simulink model "model_sim_CHBjt7"  (R2023b)
settings: Solver=ode3  StartTime=0.0  StopTime=5  FixedStep=01e-6  RelTol=1e-3
InitFcn:
  | sysinit
values from neighbouring files (symbols this model uses):
  C = 0.0234    [sysinit.m]
  f_m = frequency_modulate_start : frequency_modulate_interval : frequency_modulate_end    [simout_chbjt_par.m]    (also in simresjt7.mat = [250 300 350 400 450 500 550 600 650 700 750 800 ... (16 ele)
  L = 0.002    [sysinit.m]
  L_1 = eps    [simout_chb_par.m]    (also in simout_chbjt_par.m; simresjt7.mat = 2.22044604925e-16)
  m = modulate_radio_start : modulate_radio_interval : modulate_radio_end    [simout_chb_par.m]
  R = 1.5    [sysinit.m]
  st = 1e-6    (= 1e-06)    [sysinit.m]
undefined symbols (not defined in the file or in its folder): f, magnitude, Td, Ts2, udc
libraries: spsSeriesRLCBranchLib x120, spsDiodeLib x45, spsIGBTLib x36, spsMeanLib x20, spsCurrentMeasurementLib x16, spsVoltageMeasurementLib x11, spsThreePhaseVIMeasurementLib x10, spsOnDelayLib x9, spsMultiWindingTransformerLib x9, spsUniversalBridgeLib x9, simulink x5, spsRMSLib x2
(part 1 of 3)
settings Model: SimulationMode=accelerator  Creator=Jhchen  LastModifiedBy=ps
settings DataIOCC: ReturnWorkspaceOutputs=off
settings DebuggingCC: RTPrefix=warning

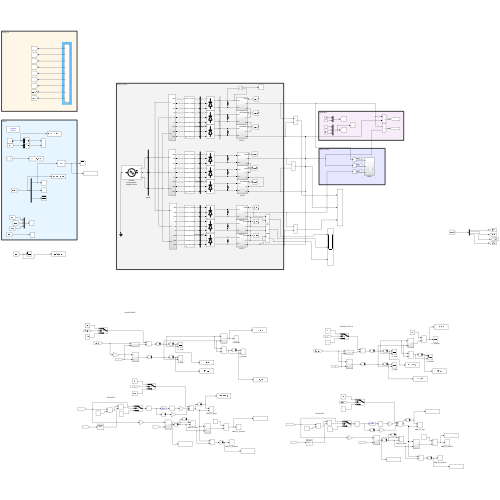
[thumbnail: Simulink's stored preview of the top-level diagram]
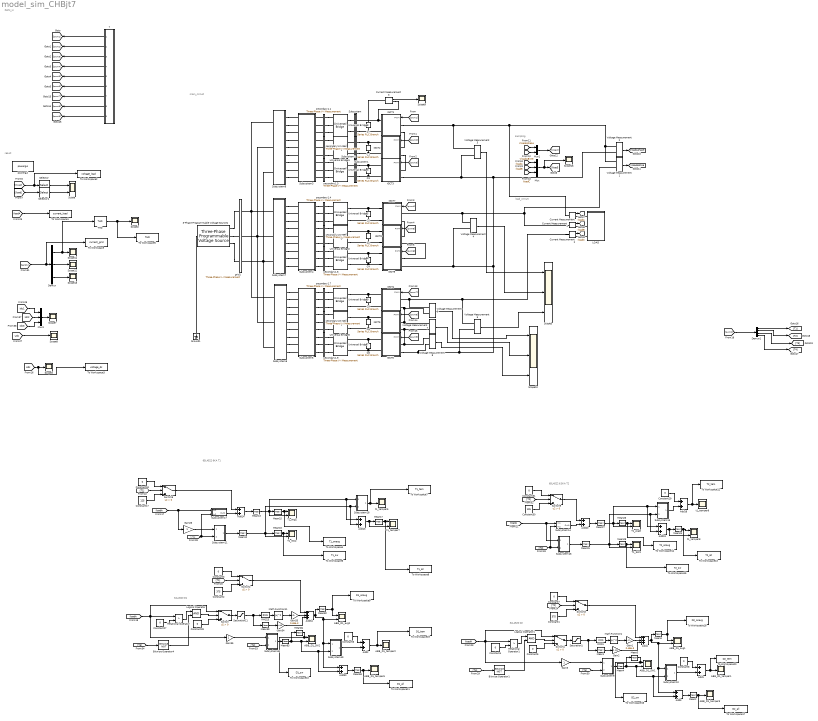
== system model_sim_CHBjt7 ==
  note: load_circuit
  note: main_circuit
  note: PWM_in
  note: result
  note: sampling
  note: 65L4522 6.5KA T2
  note: 34L4520 D1
  note: 34L4520 D2
  note: 65L4522 6KA T1
  3-Phase Programmable Voltage Source1 : spsThreePhaseProgrammableVoltageSourceLib/Three-Phase Programmable Voltage Source  PositiveSequence=[10000 0 50]  VariationEntity=None  VariationType=Step  VariationTypeAlt=Step  VariationStep=0.5  VariationRate=10  VariationMagnitude=0.3  VariationFrequency=2  VariationTiming=[0.05 1]  VariationPhaseA=off  Amplitudes=[1 0.8 1.2 1.0]  TimeValues=[0 0.1 0.15 0.2]  HarmonicGeneration=off  HarmonicA=[5 0.08 -45 2]  HarmonicB=[2 0 0 2]  Timing="[0.1  1]"  BusType=swing  Pref=0  Qref=0  Qmin=-inf  Qmax=inf
  7 : Subsystem  mask{m=m, f=f, f_car=f_m, tt=1/6, ttd=Td}
      mask prompts: m "m_p"; f "f_module"; f_car "f_carrier"; tt "ts"; ttd "td"
      mask DialogControl ParameterGroupVar Prompt: 参数
  ABB_D1_SW1 : Scope  NumInputPorts=2
  ABB_D1_SW2 : Scope  NumInputPorts=2
  ABB_D1_avg1 : Scope  NumInputPorts=2
  ABB_D1_avg2 : Scope  NumInputPorts=2
  ABB_D1_temper{1..3,6} (4 alike) : Scope
  Add{1..3,13..14,18..20,30} (9 alike) : Sum
  Add34 : Sum  Inputs=+++
  Add4 : Sum  Inputs=+++
  Bitwise Operator1 : simulink/Logic and Bit Operations/Bitwise Operator  logicop=NOT  UseBitMask=off  BitMask=bin2dec('11011001')  BitMaskRealWorld=Stored Integer
  Bitwise Operator4 : simulink/Logic and Bit Operations/Bitwise Operator  logicop=NOT  UseBitMask=off  BitMask=bin2dec('11011001')  BitMaskRealWorld=Stored Integer
  C{1..9} (9 alike) : spsSeriesRLCBranchLib/Series RLC Branch  LConnTagsString=__new0  RConnTagsString=__new0  BranchType=C  Resistance=0.0001  Inductance=1.0  SetiL0=off  InitialCurrent=0  Capacitance=C  Setx0=on  InitialVoltage=2500  Measurements=None
  Constant1 : Constant  Value=375
  Constant17 : Constant  Value=125
  Constant{3..8,18,27..29,31} (11 alike) : Constant  Value=0
  Constant2 : Constant  Value=375
  Constant30 : Constant  Value=125
  Current Measurement{,1..3} (4 alike) : spsCurrentMeasurementLib/Current Measurement  PhasorSimulation=off  OutputType=Complex  PSBequivalent=0
  Demux : Demux  Outputs=3
  Demux1 : Demux
  Gain1 : Gain  Gain=0.48e-3
  Gain2 : Gain  Gain=1.46
  Gain26 : Gain
  Gain3 : Gain
  Gain33 : Gain  Gain=0.48e-3
  Gain34 : Gain  Gain=1.46
  Gain35 : Gain
  Ground1 : spsGroundLib/Ground  LConnTagsString=a
  IGCT1 : Subsystem
      settings: PortSchema="{\"entries\":[{\"content\":{\"sides\":[{\"content\":{\"connectorIds\":[\"LConn1\",\"LConn2\"]},\"type\":\"ConnectorPlacement.EquallySpacedRectSide\",\"uuid\":\"ec2238c1-da6e-4f08-8e06-b91b3c8bb0b0\"},{\"content\":{\"connectorIds\":[\"In1\",\"RConn1\",\"RConn2\"],\"side\":\"RIGHT\"},\"type\":\"ConnectorPlacement.EquallySpacedRectSide\",\"uuid\":\"af4a6234-d788-4c0c-860c-0b54063c99a4\"},{\"content\":{\"side\":\"TOP\"},\"type\":\"ConnectorPlacement.EquallySpacedRectSide\",\"uuid\":\"bf1fb326-f044-4e19-8b18-e29d3f1aca1e\"}]},\"type\":\"ConnectorPlacement.EquallySpacedConnector\",\"uuid\":\"a6b09d66-dd31-49c2-be1b-fba678cdcd99\"}],\"packageUris\":[\"http://schema.mathworks.com/mf0/Connector/R2020b\"],\"version\":\"1.0\"}"
  IGCT2 : Subsystem
      settings: PortSchema="{\"entries\":[{\"content\":{\"sides\":[{\"content\":{\"connectorIds\":[\"LConn1\",\"LConn2\"]},\"type\":\"ConnectorPlacement.EquallySpacedRectSide\",\"uuid\":\"3b5227fd-32cc-4097-9a6a-2909540651e9\"},{\"content\":{\"connectorIds\":[\"In1\",\"RConn1\",\"RConn2\"],\"side\":\"RIGHT\"},\"type\":\"ConnectorPlacement.EquallySpacedRectSide\",\"uuid\":\"b0068562-9d9a-456b-acd2-db870c5bcace\"},{\"content\":{\"side\":\"TOP\"},\"type\":\"ConnectorPlacement.EquallySpacedRectSide\",\"uuid\":\"bbecbe08-a8e7-4703-9f6f-443f87d924da\"}]},\"type\":\"ConnectorPlacement.EquallySpacedConnector\",\"uuid\":\"6ec83c7b-e3bb-4502-bc8f-4da9ff103a20\"}],\"packageUris\":[\"http://schema.mathworks.com/mf0/Connector/R2020b\"],\"version\":\"1.0\"}"
  IGCT3 : Subsystem
      settings: PortSchema="{\"entries\":[{\"content\":{\"sides\":[{\"content\":{\"connectorIds\":[\"LConn1\",\"LConn2\"]},\"type\":\"ConnectorPlacement.EquallySpacedRectSide\",\"uuid\":\"3b5227fd-32cc-4097-9a6a-2909540651e9\"},{\"content\":{\"connectorIds\":[\"In1\",\"RConn1\",\"RConn2\"],\"side\":\"RIGHT\"},\"type\":\"ConnectorPlacement.EquallySpacedRectSide\",\"uuid\":\"b0068562-9d9a-456b-acd2-db870c5bcace\"},{\"content\":{\"side\":\"TOP\"},\"type\":\"ConnectorPlacement.EquallySpacedRectSide\",\"uuid\":\"bbecbe08-a8e7-4703-9f6f-443f87d924da\"}]},\"type\":\"ConnectorPlacement.EquallySpacedConnector\",\"uuid\":\"6ec83c7b-e3bb-4502-bc8f-4da9ff103a20\"}],\"packageUris\":[\"http://schema.mathworks.com/mf0/Connector/R2020b\"],\"version\":\"1.0\"}"
  IGCT4 : Subsystem
      settings: PortSchema="{\"entries\":[{\"content\":{\"sides\":[{\"content\":{\"connectorIds\":[\"LConn1\",\"LConn2\"]},\"type\":\"ConnectorPlacement.EquallySpacedRectSide\",\"uuid\":\"ec2238c1-da6e-4f08-8e06-b91b3c8bb0b0\"},{\"content\":{\"connectorIds\":[\"In1\",\"RConn1\",\"RConn2\"],\"side\":\"RIGHT\"},\"type\":\"ConnectorPlacement.EquallySpacedRectSide\",\"uuid\":\"af4a6234-d788-4c0c-860c-0b54063c99a4\"},{\"content\":{\"side\":\"TOP\"},\"type\":\"ConnectorPlacement.EquallySpacedRectSide\",\"uuid\":\"bf1fb326-f044-4e19-8b18-e29d3f1aca1e\"}]},\"type\":\"ConnectorPlacement.EquallySpacedConnector\",\"uuid\":\"a6b09d66-dd31-49c2-be1b-fba678cdcd99\"}],\"packageUris\":[\"http://schema.mathworks.com/mf0/Connector/R2020b\"],\"version\":\"1.0\"}"
  IGCT5 : Subsystem
      settings: PortSchema="{\"entries\":[{\"content\":{\"sides\":[{\"content\":{\"connectorIds\":[\"LConn1\",\"LConn2\"]},\"type\":\"ConnectorPlacement.EquallySpacedRectSide\",\"uuid\":\"3b5227fd-32cc-4097-9a6a-2909540651e9\"},{\"content\":{\"connectorIds\":[\"In1\",\"RConn1\",\"RConn2\"],\"side\":\"RIGHT\"},\"type\":\"ConnectorPlacement.EquallySpacedRectSide\",\"uuid\":\"b0068562-9d9a-456b-acd2-db870c5bcace\"},{\"content\":{\"side\":\"TOP\"},\"type\":\"ConnectorPlacement.EquallySpacedRectSide\",\"uuid\":\"bbecbe08-a8e7-4703-9f6f-443f87d924da\"}]},\"type\":\"ConnectorPlacement.EquallySpacedConnector\",\"uuid\":\"6ec83c7b-e3bb-4502-bc8f-4da9ff103a20\"}],\"packageUris\":[\"http://schema.mathworks.com/mf0/Connector/R2020b\"],\"version\":\"1.0\"}"
  IGCT6 : Subsystem
      settings: PortSchema="{\"entries\":[{\"content\":{\"sides\":[{\"content\":{\"connectorIds\":[\"LConn1\",\"LConn2\"]},\"type\":\"ConnectorPlacement.EquallySpacedRectSide\",\"uuid\":\"3b5227fd-32cc-4097-9a6a-2909540651e9\"},{\"content\":{\"connectorIds\":[\"In1\",\"RConn1\",\"RConn2\"],\"side\":\"RIGHT\"},\"type\":\"ConnectorPlacement.EquallySpacedRectSide\",\"uuid\":\"b0068562-9d9a-456b-acd2-db870c5bcace\"},{\"content\":{\"side\":\"TOP\"},\"type\":\"ConnectorPlacement.EquallySpacedRectSide\",\"uuid\":\"bbecbe08-a8e7-4703-9f6f-443f87d924da\"}]},\"type\":\"ConnectorPlacement.EquallySpacedConnector\",\"uuid\":\"6ec83c7b-e3bb-4502-bc8f-4da9ff103a20\"}],\"packageUris\":[\"http://schema.mathworks.com/mf0/Connector/R2020b\"],\"version\":\"1.0\"}"
  IGCT7 : Subsystem
      settings: PortSchema="{\"entries\":[{\"content\":{\"sides\":[{\"content\":{\"connectorIds\":[\"LConn1\",\"LConn2\"]},\"type\":\"ConnectorPlacement.EquallySpacedRectSide\",\"uuid\":\"ec2238c1-da6e-4f08-8e06-b91b3c8bb0b0\"},{\"content\":{\"connectorIds\":[\"In1\",\"RConn1\",\"RConn2\"],\"side\":\"RIGHT\"},\"type\":\"ConnectorPlacement.EquallySpacedRectSide\",\"uuid\":\"af4a6234-d788-4c0c-860c-0b54063c99a4\"},{\"content\":{\"side\":\"TOP\"},\"type\":\"ConnectorPlacement.EquallySpacedRectSide\",\"uuid\":\"bf1fb326-f044-4e19-8b18-e29d3f1aca1e\"}]},\"type\":\"ConnectorPlacement.EquallySpacedConnector\",\"uuid\":\"a6b09d66-dd31-49c2-be1b-fba678cdcd99\"}],\"packageUris\":[\"http://schema.mathworks.com/mf0/Connector/R2020b\"],\"version\":\"1.0\"}"
  IGCT8 : Subsystem
      settings: PortSchema="{\"entries\":[{\"content\":{\"sides\":[{\"content\":{\"connectorIds\":[\"LConn1\",\"LConn2\"]},\"type\":\"ConnectorPlacement.EquallySpacedRectSide\",\"uuid\":\"3b5227fd-32cc-4097-9a6a-2909540651e9\"},{\"content\":{\"connectorIds\":[\"In1\",\"RConn1\",\"RConn2\"],\"side\":\"RIGHT\"},\"type\":\"ConnectorPlacement.EquallySpacedRectSide\",\"uuid\":\"b0068562-9d9a-456b-acd2-db870c5bcace\"},{\"content\":{\"side\":\"TOP\"},\"type\":\"ConnectorPlacement.EquallySpacedRectSide\",\"uuid\":\"bbecbe08-a8e7-4703-9f6f-443f87d924da\"}]},\"type\":\"ConnectorPlacement.EquallySpacedConnector\",\"uuid\":\"6ec83c7b-e3bb-4502-bc8f-4da9ff103a20\"}],\"packageUris\":[\"http://schema.mathworks.com/mf0/Connector/R2020b\"],\"version\":\"1.0\"}"
  IGCT9 : Subsystem
      settings: PortSchema="{\"entries\":[{\"content\":{\"sides\":[{\"content\":{\"connectorIds\":[\"LConn1\",\"LConn2\"]},\"type\":\"ConnectorPlacement.EquallySpacedRectSide\",\"uuid\":\"3b5227fd-32cc-4097-9a6a-2909540651e9\"},{\"content\":{\"connectorIds\":[\"In1\",\"RConn1\",\"RConn2\"],\"side\":\"RIGHT\"},\"type\":\"ConnectorPlacement.EquallySpacedRectSide\",\"uuid\":\"b0068562-9d9a-456b-acd2-db870c5bcace\"},{\"content\":{\"side\":\"TOP\"},\"type\":\"ConnectorPlacement.EquallySpacedRectSide\",\"uuid\":\"bbecbe08-a8e7-4703-9f6f-443f87d924da\"}]},\"type\":\"ConnectorPlacement.EquallySpacedConnector\",\"uuid\":\"6ec83c7b-e3bb-4502-bc8f-4da9ff103a20\"}],\"packageUris\":[\"http://schema.mathworks.com/mf0/Connector/R2020b\"],\"version\":\"1.0\"}"
  LOAD : Subsystem
  Logical Operator : Logic  AllPortsSameDT=off  OutDataTypeStr=boolean
  Logical Operator1 : Logic  AllPortsSameDT=off  OutDataTypeStr=boolean
  Math Function1 : Math  Operator=magnitude^2  SignedPower=on
  Math Function11 : Math  Operator=magnitude^2  SignedPower=on
  Mean{1,4,12..13,25,27,39,83} (8 alike) : spsMeanLib/Mean  Freq=2000  Vinit=0  Ts=1e-6
  Mean{15..16,26,28} (4 alike) : spsMeanLib/Mean  Freq=f  Vinit=0  Ts=Ts2
  Mean{2..3,5,17,24,58,82,84} (8 alike) : spsMeanLib/Mean  Freq=f  Vinit=0  Ts=1e-6
  Mux : Mux  Inputs=3
  Mux1 : Mux  Inputs=2
  Mux3 : Mux  Inputs=3
  RMS1 : spsRMSLib/RMS  TrueRMS=on  Freq=2000  RMSInit=0  Ts=1e-6
  RMS23 : spsRMSLib/RMS  TrueRMS=on  Freq=2000  RMSInit=0  Ts=1e-6
  Relational Operator : RelationalOperator  Operator=>  OutDataTypeStr=boolean  RndMeth=Simplest  InputSameDT=off
  Relational Operator1 : RelationalOperator  Operator=>  OutDataTypeStr=boolean  RndMeth=Simplest  InputSameDT=off
  Saturation1 : Saturate  UpperLimit=5500  LowerLimit=0
  Saturation11 : Saturate  UpperLimit=5500  LowerLimit=0
  Scope : Scope  NumInputPorts=2
  Scope10 : Scope  NumInputPorts=3
  Scope{2..3,7..9,11..13,16} (9 alike) : Scope
  Scope5 : Scope  NumInputPorts=3
  Selector : Selector  InputPortWidth=2  IndexOptions=Index vector (dialog)  Indices=[1]  OutputSizes=1
  Selector1 : Selector  InputPortWidth=3  IndexOptions=Index vector (dialog)  Indices=[1]  OutputSizes=1
  Subsystem : Subsystem
  Subsystem1 : Subsystem
  Subsystem10 : Subsystem
  Subsystem11 : Subsystem
  Subsystem14 : Subsystem
  Subsystem15 : Subsystem
  Subsystem16 : Subsystem
  Subsystem17 : Subsystem
  Subsystem18 : Subsystem
  Subsystem2 : Subsystem
  Subsystem3 : Subsystem  mask{L_in=L_1}
      mask prompts: L_in "L"
      mask DialogControl ParameterGroupVar Prompt: 参数
  Subsystem4 : Subsystem  mask{L_in=L_1}
      mask prompts: L_in "L"
      mask DialogControl ParameterGroupVar Prompt: 参数
  Subsystem48 : Subsystem
  Subsystem49 : Subsystem
  Subsystem5 : Subsystem  mask{L_in=L_1}
      mask prompts: L_in "L"
      mask DialogControl ParameterGroupVar Prompt: 参数
  Subsystem6 : Subsystem
  Subsystem7 : Subsystem
  Subsystem8 : Subsystem
  Subsystem9 : Subsystem
  Switch{,1..3,6,9} (6 alike) : Switch  Criteria=u2 > Threshold  SaturateOnIntegerOverflow=off  InputSameDT=off
  T1_SW2 : Scope  NumInputPorts=2
  T1_SW3 : Scope  NumInputPorts=2
  T1_avg2 : Scope  NumInputPorts=2
  T1_avg3 : Scope  NumInputPorts=2
  THD : spsTHDLib/THD  Freq=50  Ts=0
  To Workspace : ToWorkspace  VariableName=current_grid  SaveFormat=Structure With Time  SampleTime=-1
  To Workspace1 : ToWorkspace  VariableName=current_load  SaveFormat=Structure With Time  SampleTime=-1
  To Workspace10 : ToWorkspace  VariableName=D1_sw  SaveFormat=Structure With Time  SampleTime=-1
  To Workspace11 : ToWorkspace  VariableName=D1_all  SaveFormat=Structure With Time  SampleTime=-1
  To Workspace12 : ToWorkspace  VariableName=T2_tem  SaveFormat=Structure With Time  SampleTime=-1
  To Workspace13 : ToWorkspace  VariableName=T2_all  SaveFormat=Structure With Time  SampleTime=-1
  To Workspace14 : ToWorkspace  VariableName=T2_onavg  SaveFormat=Structure With Time  SampleTime=-1
  To Workspace15 : ToWorkspace  VariableName=T2_sw  SaveFormat=Structure With Time  SampleTime=-1
  To Workspace16 : ToWorkspace  VariableName=D2_sw  SaveFormat=Structure With Time  SampleTime=-1
  To Workspace17 : ToWorkspace  VariableName=D2_all  SaveFormat=Structure With Time  SampleTime=-1
  To Workspace18 : ToWorkspace  VariableName=D2_onavg  SaveFormat=Structure With Time  SampleTime=-1
  To Workspace19 : ToWorkspace  VariableName=D1_tem  SaveFormat=Structure With Time  SampleTime=-1
  To Workspace2 : ToWorkspace  VariableName=voltage_load  SaveFormat=Structure With Time  SampleTime=-1
  To Workspace20 : ToWorkspace  VariableName=D2_tem  SaveFormat=Structure With Time  SampleTime=-1
  To Workspace3 : ToWorkspace  VariableName=voltage_dc  SaveFormat=Structure With Time  SampleTime=-1
  To Workspace4 : ToWorkspace  VariableName=T1_onavg  SaveFormat=Structure With Time  SampleTime=-1
  To Workspace5 : ToWorkspace  VariableName=THD  SaveFormat=Structure With Time  SampleTime=-1
  To Workspace6 : ToWorkspace  VariableName=T1_sw  SaveFormat=Structure With Time  SampleTime=-1
  To Workspace7 : ToWorkspace  VariableName=T1_tem  SaveFormat=Structure With Time  SampleTime=-1
  To Workspace8 : ToWorkspace  VariableName=T1_all  SaveFormat=Structure With Time  SampleTime=-1
  To Workspace9 : ToWorkspace  VariableName=D1_onavg  SaveFormat=Structure With Time  SampleTime=-1
  Universal Bridge{1..9} (9 alike) : spsUniversalBridgeLib/Universal Bridge  Arms=3  SnubberResistance=1e5  SnubberCapacitance=inf  Device=Diodes  Ron=1e-3  Lon=0  ForwardVoltages="[  0  0  ]"  ForwardVoltage=0  GTOparameters=[ 10e-6 , 20e-6 ]  IGBTparameters=[ 1e-6 , 2e-6 ]  Measurements=None  Measurements_2=None  converterType=Rectifier
  Voltage Measurement{1..8} (8 alike) : spsVoltageMeasurementLib/Voltage Measurement  PhasorSimulation=off  OutputType=Complex  PSBequivalent=0
  grid1 : spsThreePhaseVIMeasurementLib/Three-Phase V-I Measurement  VoltageMeasurement=phase-to-ground  SetLabelV=on  LabelV=Vgrid1  Vpu=off  VpuLL=off  CurrentMeasurement=yes  SetLabelI=on  LabelI=Igrid1  Ipu=off  Pbase=1e3  Vbase=380  OutputType=Magnitude  PhasorSimulation=off  PSBequivalent=0
  powergui : spspowerguiLib/powergui  Priority=1  SimulationMode=Discrete  SampleTime=st  frequency=60  Iterations=50  frequencyindice=50  Pbase=100e6  ErrMax=1e-4  UnitsV=kV  UnitsW=MW  buscounter=0  FunctionMessages=off  echomessages=off  EnableUseOfTLC=off  CurrentSourceSwitches=off  DisableSnubberDevices=off  DisableRonSwitches=off  DisableVfSwitches=off  DisplayEquations=off  AutomaticDiscreteSolvers=off  SolverType=Tustin/Backward Euler (TBE)  Interpol=off  ExternalGateDelay=off  methode=off  Ts=100  x0status=blocks  SPID=on  SwTol=0  HookPort=off  NonlinearTolerance=1e-4  nMaxIteration=100  ContinueOnMaxIteration=off  RestoreLinks=warning  ResistiveCurrentMeasurement=off  Frange=[0:2:500]  Ylog=off  Xlog=on  ShowGrid=off  save=off  variable=ZData  structure=0  ZoomFFT=off  StartTime=0.0  cycles=1  DisplayStyle=1  fundamental=60  FreqAxis=off  MaxFrequency=1000  frequencyindicesteady=1  RmsSteady=1  display=off
  secondary1.1 : spsThreePhaseVIMeasurementLib/Three-Phase V-I Measurement  VoltageMeasurement=phase-to-phase  SetLabelV=on  LabelV=Vsecondary_a1  Vpu=off  VpuLL=off  CurrentMeasurement=yes  SetLabelI=on  LabelI=Isecondary_a1  Ipu=off  Pbase=1e3  Vbase=380  OutputType=Magnitude  PhasorSimulation=off  PSBequivalent=0
  secondary1.2 : spsThreePhaseVIMeasurementLib/Three-Phase V-I Measurement  VoltageMeasurement=phase-to-phase  SetLabelV=on  LabelV=Vsecondary_a2  Vpu=off  VpuLL=off  CurrentMeasurement=yes  SetLabelI=on  LabelI=Isecondary_a2  Ipu=off  Pbase=1e3  Vbase=380  OutputType=Magnitude  PhasorSimulation=off  PSBequivalent=0
  secondary1.3 : spsThreePhaseVIMeasurementLib/Three-Phase V-I Measurement  VoltageMeasurement=phase-to-phase  SetLabelV=on  LabelV=Vsecondary_a3  Vpu=off  VpuLL=off  CurrentMeasurement=yes  SetLabelI=on  LabelI=Isecondary_a3  Ipu=off  Pbase=1e3  Vbase=380  OutputType=Magnitude  PhasorSimulation=off  PSBequivalent=0
  secondary1.4 : spsThreePhaseVIMeasurementLib/Three-Phase V-I Measurement  VoltageMeasurement=phase-to-phase  SetLabelV=on  LabelV=Vsecondary_a4  Vpu=off  VpuLL=off  CurrentMeasurement=yes  SetLabelI=on  LabelI=Isecondary_a4  Ipu=off  Pbase=1e3  Vbase=380  OutputType=Magnitude  PhasorSimulation=off  PSBequivalent=0
  secondary1.5 : spsThreePhaseVIMeasurementLib/Three-Phase V-I Measurement  VoltageMeasurement=phase-to-phase  SetLabelV=on  LabelV=Vsecondary_a5  Vpu=off  VpuLL=off  CurrentMeasurement=yes  SetLabelI=on  LabelI=Isecondary_a5  Ipu=off  Pbase=1e3  Vbase=380  OutputType=Magnitude  PhasorSimulation=off  PSBequivalent=0
  secondary1.6 : spsThreePhaseVIMeasurementLib/Three-Phase V-I Measurement  VoltageMeasurement=phase-to-phase  SetLabelV=on  LabelV=Vsecondary_a6  Vpu=off  VpuLL=off  CurrentMeasurement=yes  SetLabelI=on  LabelI=Isecondary_a6  Ipu=off  Pbase=1e3  Vbase=380  OutputType=Magnitude  PhasorSimulation=off  PSBequivalent=0
  secondary1.7 : spsThreePhaseVIMeasurementLib/Three-Phase V-I Measurement  VoltageMeasurement=phase-to-phase  SetLabelV=on  LabelV=Vsecondary_a7  Vpu=off  VpuLL=off  CurrentMeasurement=yes  SetLabelI=on  LabelI=Isecondary_a7  Ipu=off  Pbase=1e3  Vbase=380  OutputType=Magnitude  PhasorSimulation=off  PSBequivalent=0
  secondary1.8 : spsThreePhaseVIMeasurementLib/Three-Phase V-I Measurement  VoltageMeasurement=phase-to-phase  SetLabelV=on  LabelV=Vsecondary_a8  Vpu=off  VpuLL=off  CurrentMeasurement=yes  SetLabelI=on  LabelI=Isecondary_a8  Ipu=off  Pbase=1e3  Vbase=380  OutputType=Magnitude  PhasorSimulation=off  PSBequivalent=0
  secondary1.9 : spsThreePhaseVIMeasurementLib/Three-Phase V-I Measurement  VoltageMeasurement=phase-to-phase  SetLabelV=on  LabelV=Vsecondary_a9  Vpu=off  VpuLL=off  CurrentMeasurement=yes  SetLabelI=on  LabelI=Isecondary_a9  Ipu=off  Pbase=1e3  Vbase=380  OutputType=Magnitude  PhasorSimulation=off  PSBequivalent=0
  t1_temper5 : Scope
  t1_temper7 : Scope  NumInputPorts=2
  t1_temper8 : Scope  NumInputPorts=2
  t1_temper9 : Scope
  tag scope: IloadA=global, IloadB=global, IloadC=global, VloadABline=global, VloadAphase=global
  wires:
  [pwm1] -> IGCT1/1(PWM)
  [Vload] -> To Workspace2/1, Selector/1
  Selector/1 -> Scope/1
  [Iload] -> Selector1/1
  Selector1/1 -> Scope/2
  Current Measurement/1 -> [IloadA]
  Current Measurement1/1 -> [IloadB]
  Current Measurement2/1 -> [IloadC]
  [IloadC] -> Mux/3
  [IloadB] -> Mux/2
  [IloadA] -> Mux/1
  Mux/1 -> Scope16/1, [Iload]
  Voltage Measurement2/1 -> [VloadAphase]
  Voltage Measurement1/1 -> [VloadABline]
  [VloadAphase] -> Mux1/1
  [VloadABline] -> Mux1/2
  Mux1/1 -> [Vload]
  [Igrid1] -> To Workspace/1, Demux/1
  [IloadA] -> To Workspace1/1
  [pwm4] -> IGCT7/1(PWM)
  [pwm5] -> IGCT8/1(PWM)
  [pwm6] -> IGCT9/1(PWM)
  [pwm7] -> IGCT4/1(PWM)
  [pwm8] -> IGCT5/1(PWM)
  [pwm9] -> IGCT6/1(PWM)
  [pwm2] -> IGCT2/1(PWM)
  [pwm3] -> IGCT3/1(PWM)
  7/1(Out1) -> [pwm1]
  7/2(Out2) -> [pwm2]
  7/3(Out3) -> [pwm3]
  7/9(Out9) -> [pwm9]
  7/8(Out8) -> [pwm8]
  7/7(Out7) -> [pwm7]
  7/6(Out6) -> [pwm6]
  7/5(Out5) -> [pwm5]
  7/4(Out4) -> [pwm4]
  Voltage Measurement5/1 -> Scope5/3
  Voltage Measurement4/1 -> Scope5/2
  Voltage Measurement3/1 -> Scope5/1
  [Udc] -> Scope8/1
  Current Measurement3/1 -> Scope9/1
  Voltage Measurement6/1 -> Scope10/1
  Voltage Measurement7/1 -> Scope10/2
  Voltage Measurement8/1 -> Scope10/3
  Demux/1 -> THD/1, Scope11/1
  Demux/3 -> Scope13/1
  Demux/2 -> Scope12/1
  [Idc1] -> Mux3/1
  [Idc2] -> Mux3/2
  [Idc3] -> Mux3/3
  Mux3/1 -> Scope7/1
  THD/1 -> To Workspace5/1, Scope2/1
  [Udc] -> To Workspace3/1, Scope3/1
  [IloadA] -> Switch/1, Gain35/1, Relational Operator/1
  Mean17/1 -> To Workspace8/1, t1_temper7/1
  Add13/1 -> t1_temper7/2, Mean17/1
  Demux1/1 -> [T1]
  Gain34/1 -> Add34/3
  Constant28/1 -> Switch/3
  Bitwise Operator4/1 -> Logical Operator/2
  Constant17/1 -> Switch6/3
  Constant2/1 -> Switch2/3
  Demux1/2 -> [T2]
  Mean16/1 -> To Workspace6/1, T1_SW2/1
  [T1] -> Switch2/2
  Add34/1 -> Add30/1, Subsystem49/1(In1), ABB_D1_avg2/2, Mean82/1
  Add20/1 -> Mean27/1
  Add19/1 -> t1_temper8/2, Mean24/1
  Gain26/1 -> Subsystem11/1(In1)
  Switch6/1 -> Add14/1
  Mean12/1 -> Subsystem18/2(In2), Add13/2, T1_SW2/2, Mean16/1
  Subsystem17/1(Out1) -> Add14/2
  Add30/1 -> Mean58/1
  Constant6/1 -> Add2/1
  Mean58/1 -> ABB_D1_temper6/1, To Workspace11/1
  Mean28/1 -> To Workspace15/1, T1_SW3/1
  [T1] -> Subsystem11/2(In2), Subsystem17/2(In2)
  [IloadA] -> Gain26/1, Subsystem17/1(In1)
  Add3/1 -> Mean2/1
  [IloadA] -> Subsystem16/1(In1), Subsystem14/1(In1)
  Mean5/1 -> ABB_D1_SW1/1, To Workspace16/1
  RMS1/1 -> Math Function1/1
  Add2/1 -> To Workspace19/1, ABB_D1_temper2/1
  Add4/1 -> Mean3/1, ABB_D1_avg1/2, Subsystem10/1(In1), Add3/1
  Relational Operator1/1 -> Logical Operator1/1
  [T2] -> Switch3/2
  Constant7/1 -> Switch3/1
  Gain1/1 -> Add4/2
  [IloadA] -> Relational Operator1/1, Gain3/1, Switch1/1
  Subsystem11/1(Out1) -> Mean12/1
  Add1/1 -> To Workspace20/1, ABB_D1_temper1/1
  Gain3/1 -> Subsystem9/1(In1)
  Mean3/1 -> To Workspace18/1, ABB_D1_avg1/1
  Demux1/3 -> [T3]
  Logical Operator1/1 -> Switch1/2
  Switch1/1 -> Saturation1/1
  Mean4/1 -> ABB_D1_SW1/2, Subsystem10/2(In2), Add3/2, Mean5/1
  Saturation1/1 -> RMS1/1, Mean1/1
  Add18/1 -> To Workspace12/1, t1_temper9/1
  Constant18/1 -> Switch6/1
  Subsystem16/1(Out1) -> Mean25/1
  Constant29/1 -> Add18/1
  [T2] -> Subsystem14/2(In2), Subsystem16/2(In2)
  Subsystem15/1(Out1) -> Add18/2
  Mean27/1 -> T1_avg3/2, Mean26/1, Subsystem15/1(In1), Add19/1
  Relational Operator/1 -> Logical Operator/1
  Subsystem14/1(Out1) -> Add20/2
  [T1] -> Switch6/2
  Constant31/1 -> Switch9/1
  Constant1/1 -> Switch3/3
  Mean24/1 -> To Workspace13/1, t1_temper8/1
  RMS23/1 -> Math Function11/1
  [T2] -> Switch9/2
  Mean84/1 -> To Workspace10/1, ABB_D1_SW2/1
  Saturation11/1 -> Mean39/1, RMS23/1
  Switch9/1 -> Add20/1
  Constant30/1 -> Switch9/3
  Constant5/1 -> Switch1/3
  Mean25/1 -> Subsystem15/2(In2), Add19/2, T1_SW3/2, Mean28/1
  Mean82/1 -> ABB_D1_avg2/1, To Workspace9/1
  Gain35/1 -> Subsystem48/1(In1)
  Math Function11/1 -> Gain33/1
  Bitwise Operator1/1 -> Logical Operator1/2
  Add14/1 -> Mean13/1
  Mean26/1 -> To Workspace14/1, T1_avg3/1
  Mean39/1 -> Gain34/1
  Switch2/1 -> Add34/1
  Constant27/1 -> Relational Operator/2
  Subsystem48/1(Out1) -> Mean83/1
  Subsystem18/1(Out1) -> To Workspace7/1, t1_temper5/1
  Mean15/1 -> To Workspace4/1, T1_avg2/1
  [T3] -> Subsystem48/2(In2)
  Demux1/4 -> [T4]
  Constant8/1 -> Add1/1
  Gain2/1 -> Add4/3
  Mean13/1 -> T1_avg2/2, Mean15/1, Subsystem18/1(In1), Add13/1
  [T3] -> Bitwise Operator4/1
  [T4] -> Subsystem9/2(In2)
  Subsystem10/1(Out1) -> Add1/2
  Math Function1/1 -> Gain1/1
  Mean2/1 -> To Workspace17/1, ABB_D1_temper3/1
  Subsystem49/1(Out1) -> Add2/2
  [T4] -> Bitwise Operator1/1
  Logical Operator/1 -> Switch/2
  Constant3/1 -> Switch2/1
  Switch/1 -> Saturation11/1
  Constant4/1 -> Relational Operator1/2
  Mean1/1 -> Gain2/1
  [pwm1] -> Demux1/1
  Mean83/1 -> Mean84/1, Add30/2, Subsystem49/2(In2), ABB_D1_SW2/2
  Switch3/1 -> Add4/1
  Subsystem9/1(Out1) -> Mean4/1
  Gain33/1 -> Add34/2
  connections:
  3-Phase Programmable Voltage Source1/RConn3 -- grid1/LConn3
  3-Phase Programmable Voltage Source1/RConn2 -- grid1/LConn2
  secondary1.1/RConn2 -- Universal Bridge8/LConn2
  secondary1.1/RConn3 -- Universal Bridge8/LConn3
  secondary1.2/RConn1 -- Universal Bridge1/LConn1
  secondary1.2/RConn2 -- Universal Bridge1/LConn2
  secondary1.2/RConn3 -- Universal Bridge1/LConn3
  secondary1.1/RConn1 -- Universal Bridge8/LConn1
  IGCT2/LConn2 -- Subsystem1/RConn2 -- C1/RConn1
  IGCT2/LConn1 -- Subsystem1/RConn1 -- C1/LConn1
  Universal Bridge8/RConn1 -- Subsystem/LConn1
  Universal Bridge8/RConn2 -- Subsystem/LConn2
  Subsystem/RConn2 -- IGCT1/LConn2 -- C7/RConn1
  IGCT1/LConn1 -- Current Measurement3/RConn1 -- Subsystem/RConn1
  IGCT1/RConn2 -- IGCT2/RConn1
  IGCT3/LConn2 -- Subsystem2/RConn2 -- C3/RConn1
  secondary1.3/RConn1 -- Universal Bridge3/LConn1
  C3/LConn1 -- Subsystem2/RConn1 -- IGCT3/LConn1
  secondary1.3/RConn3 -- Universal Bridge3/LConn3
  secondary1.3/RConn2 -- Universal Bridge3/LConn2
  3-Phase Programmable Voltage Source1/RConn1 -- grid1/LConn1
  LOAD/LConn2 -- Current Measurement1/RConn1
  Current Measurement/RConn1 -- LOAD/LConn1
  Current Measurement2/RConn1 -- LOAD/LConn3
  Ground1/LConn1 -- 3-Phase Programmable Voltage Source1/LConn1
  IGCT2/RConn2 -- IGCT3/RConn1
  IGCT6/RConn2 -- Voltage Measurement8/LConn2 -- Voltage Measurement5/LConn2 -- Voltage Measurement3/LConn2 -- IGCT3/RConn2 -- Voltage Measurement2/LConn2 -- Voltage Measurement4/LConn2 -- IGCT9/RConn2
  C5/LConn1 -- IGCT7/LConn1 -- Universal Bridge5/RConn1
  C5/RConn1 -- IGCT7/LConn2 -- Universal Bridge5/RConn2
  C4/LConn1 -- IGCT9/LConn1 -- Universal Bridge4/RConn1
  Universal Bridge4/RConn2 -- IGCT9/LConn2 -- C4/RConn1
  Universal Bridge2/RConn2 -- IGCT8/LConn2 -- C2/RConn1
  Universal Bridge2/RConn1 -- IGCT8/LConn1 -- C2/LConn1
  secondary1.6/RConn2 -- Universal Bridge4/LConn2
  secondary1.4/RConn3 -- Universal Bridge5/LConn3
  IGCT9/RConn1 -- IGCT8/RConn2
  secondary1.5/RConn1 -- Universal Bridge2/LConn1
  secondary1.6/RConn3 -- Universal Bridge4/LConn3
  IGCT8/RConn1 -- IGCT7/RConn2
  secondary1.4/RConn2 -- Universal Bridge5/LConn2
  secondary1.4/RConn1 -- Universal Bridge5/LConn1
  secondary1.5/RConn3 -- Universal Bridge2/LConn3
  secondary1.6/RConn1 -- Universal Bridge4/LConn1
  secondary1.5/RConn2 -- Universal Bridge2/LConn2
  C9/LConn1 -- IGCT4/LConn1 -- Universal Bridge9/RConn1
  C9/RConn1 -- IGCT4/LConn2 -- Universal Bridge9/RConn2
  C8/LConn1 -- IGCT6/LConn1 -- Universal Bridge7/RConn1
  Universal Bridge7/RConn2 -- IGCT6/LConn2 -- C8/RConn1
  Universal Bridge6/RConn2 -- IGCT5/LConn2 -- C6/RConn1
  Universal Bridge6/RConn1 -- IGCT5/LConn1 -- C6/LConn1
  secondary1.9/RConn2 -- Universal Bridge7/LConn2
  secondary1.7/RConn3 -- Universal Bridge9/LConn3
  IGCT5/RConn2 -- Voltage Measurement7/LConn2 -- Voltage Measurement8/LConn1 -- IGCT6/RConn1
  secondary1.8/RConn1 -- Universal Bridge6/LConn1
  secondary1.9/RConn3 -- Universal Bridge7/LConn3
  IGCT5/RConn1 -- Voltage Measurement7/LConn1 -- Voltage Measurement6/LConn2 -- IGCT4/RConn2
  secondary1.7/RConn2 -- Universal Bridge9/LConn2
  secondary1.7/RConn1 -- Universal Bridge9/LConn1
  secondary1.8/RConn3 -- Universal Bridge6/LConn3
  secondary1.9/RConn1 -- Universal Bridge7/LConn1
  secondary1.8/RConn2 -- Universal Bridge6/LConn2
  IGCT1/RConn1 -- Voltage Measurement3/LConn1 -- Voltage Measurement1/LConn1 -- Voltage Measurement2/LConn1 -- Current Measurement/LConn1
  Voltage Measurement1/LConn2 -- Current Measurement1/LConn1 -- Voltage Measurement4/LConn1 -- IGCT7/RConn1
  Current Measurement2/LConn1 -- Voltage Measurement5/LConn1 -- Voltage Measurement6/LConn1 -- IGCT4/RConn1
  Current Measurement3/LConn1 -- C7/LConn1
  Subsystem1/LConn1 -- Universal Bridge1/RConn1
  Subsystem1/LConn2 -- Universal Bridge1/RConn2
  Subsystem2/LConn1 -- Universal Bridge3/RConn1
  Subsystem2/LConn2 -- Universal Bridge3/RConn2
  Subsystem8/LConn1 -- Subsystem7/LConn1 -- Subsystem6/LConn1 -- grid1/RConn1
  Subsystem8/LConn2 -- grid1/RConn2 -- Subsystem7/LConn2 -- Subsystem6/LConn2
  Subsystem8/LConn3 -- grid1/RConn3 -- Subsystem7/LConn3 -- Subsystem6/LConn3
  Subsystem8/RConn1 -- Subsystem3/LConn1
  Subsystem8/RConn2 -- Subsystem3/LConn2
  Subsystem8/RConn3 -- Subsystem3/LConn3
  Subsystem8/RConn4 -- Subsystem3/LConn4
  Subsystem8/RConn5 -- Subsystem3/LConn5
  Subsystem8/RConn6 -- Subsystem3/LConn6
  Subsystem8/RConn7 -- Subsystem3/LConn7
  Subsystem8/RConn8 -- Subsystem3/LConn8
  Subsystem8/RConn9 -- Subsystem3/LConn9
  secondary1.1/LConn1 -- Subsystem3/RConn1
  secondary1.1/LConn2 -- Subsystem3/RConn2
  secondary1.1/LConn3 -- Subsystem3/RConn3
  secondary1.2/LConn1 -- Subsystem3/RConn4
  secondary1.2/LConn2 -- Subsystem3/RConn5
  secondary1.2/LConn3 -- Subsystem3/RConn6
  secondary1.3/LConn1 -- Subsystem3/RConn7
  secondary1.3/LConn2 -- Subsystem3/RConn8
  secondary1.3/LConn3 -- Subsystem3/RConn9
  Subsystem6/RConn1 -- Subsystem5/LConn1
  Subsystem6/RConn2 -- Subsystem5/LConn2
  Subsystem6/RConn3 -- Subsystem5/LConn3
  Subsystem6/RConn4 -- Subsystem5/LConn4
  Subsystem6/RConn5 -- Subsystem5/LConn5
  Subsystem6/RConn6 -- Subsystem5/LConn6
  Subsystem6/RConn7 -- Subsystem5/LConn7
  Subsystem6/RConn8 -- Subsystem5/LConn8
  Subsystem6/RConn9 -- Subsystem5/LConn9
  Subsystem5/RConn1 -- secondary1.7/LConn1
  Subsystem5/RConn2 -- secondary1.7/LConn2
  Subsystem5/RConn3 -- secondary1.7/LConn3
  Subsystem5/RConn4 -- secondary1.8/LConn1
  Subsystem5/RConn5 -- secondary1.8/LConn2
  Subsystem5/RConn6 -- secondary1.8/LConn3
  Subsystem5/RConn7 -- secondary1.9/LConn1
  Subsystem5/RConn8 -- secondary1.9/LConn2
  Subsystem5/RConn9 -- secondary1.9/LConn3
  Subsystem4/RConn1 -- secondary1.4/LConn1
  Subsystem4/RConn2 -- secondary1.4/LConn2
  Subsystem4/RConn3 -- secondary1.4/LConn3
  Subsystem4/RConn4 -- secondary1.5/LConn1
  Subsystem4/RConn5 -- secondary1.5/LConn2
  Subsystem4/RConn6 -- secondary1.5/LConn3
  Subsystem4/RConn7 -- secondary1.6/LConn1
  Subsystem4/RConn8 -- secondary1.6/LConn2
  Subsystem4/RConn9 -- secondary1.6/LConn3
  Subsystem7/RConn1 -- Subsystem4/LConn1
  Subsystem7/RConn2 -- Subsystem4/LConn2
  Subsystem7/RConn3 -- Subsystem4/LConn3
  Subsystem7/RConn4 -- Subsystem4/LConn4
  Subsystem7/RConn5 -- Subsystem4/LConn5
  Subsystem7/RConn6 -- Subsystem4/LConn6
  Subsystem7/RConn7 -- Subsystem4/LConn7
  Subsystem7/RConn8 -- Subsystem4/LConn8
  Subsystem7/RConn9 -- Subsystem4/LConn9

== system model_sim_CHBjt7/7 ==
  2/3*pi : Subsystem
  2/3*pi1 : Subsystem
  2/3*pi2 : Subsystem
  Scope : Scope  NumInputPorts=3
  Sine Wave : Sin  Amplitude=m*1000  Frequency=f*2*pi  Phase=2/3*pi  SampleTime=0
  Sine Wave1 : Sin  Amplitude=m*1000  Frequency=f*2*pi  SampleTime=0
  Sine Wave2 : Sin  Amplitude=m*1000  Frequency=f*2*pi  Phase=-2/3*pi  SampleTime=0
  Subsystem : Subsystem
  Out1 : Outport
  Out2 : Outport  Port=2
  Out3 : Outport  Port=3
  Out4 : Outport  Port=4
  Out5 : Outport  Port=5
  Out6 : Outport  Port=6
  Out7 : Outport  Port=7
  Out8 : Outport  Port=8
  Out9 : Outport  Port=9
  wires:
  2/3*pi1/2(Out2) -> Out5/1
  2/3*pi/2(Out2) -> Out2/1
  2/3*pi/3(Out3) -> Out3/1
  2/3*pi/1(Out1) -> Out1/1
  2/3*pi2/2(Out2) -> Out8/1
  2/3*pi1/1(Out1) -> Out4/1
  2/3*pi1/3(Out3) -> Out6/1
  2/3*pi2/1(Out1) -> Out7/1
  2/3*pi2/3(Out3) -> Out9/1
  Sine Wave/1 -> Subsystem/1(In1)
  Sine Wave1/1 -> Subsystem/2(In2)
  Sine Wave2/1 -> Subsystem/3(In3)
  Subsystem/1(Out1) -> Scope/1, 2/3*pi/1(In1)
  Subsystem/2(Out2) -> 2/3*pi1/1(In1), Scope/2
  Subsystem/3(Out3) -> 2/3*pi2/1(In1), Scope/3

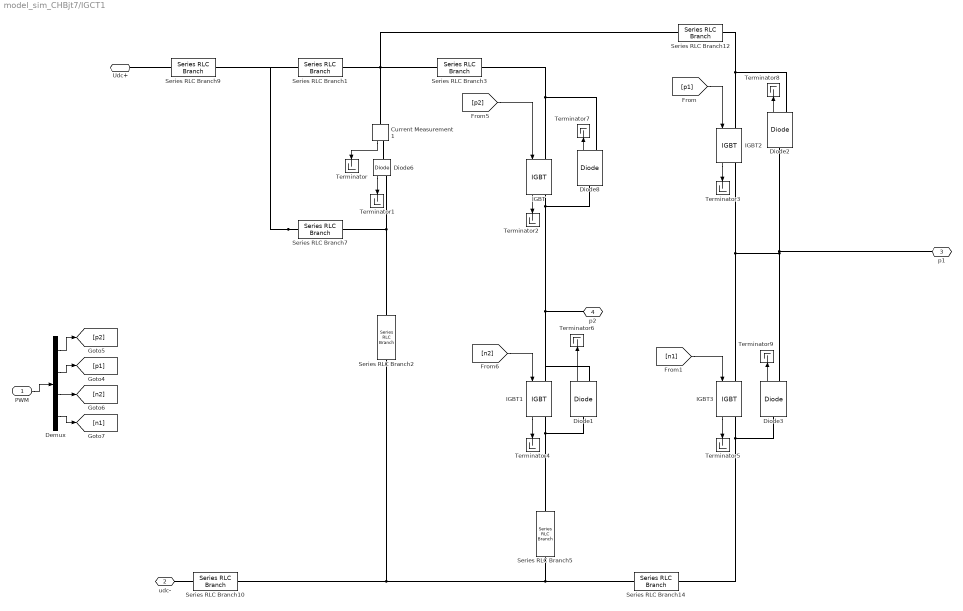
== system model_sim_CHBjt7/IGCT1 ==
  PWM : Inport
  Current Measurement1 : spsCurrentMeasurementLib/Current Measurement  PhasorSimulation=off  OutputType=Complex  PSBequivalent=0
  Demux : Demux
  Diode{1..3,6,8} (5 alike) : spsDiodeLib/Diode  Ron=rto  Lon=0  Vf=vto  IC=0  UseSnubber=off  Rs=500  Cs=250e-9  Measurements=on
  IGBT{,1..3} (4 alike) : spsIGBTLib/IGBT  Ron=rt  Lon=0  Vf=vt  Tf=1e-6  Tt=2e-6  IC=0  Rs=1e5  Cs=inf  Measurements=on
  Series RLC Branch1 : spsSeriesRLCBranchLib/Series RLC Branch  LConnTagsString=__new0  RConnTagsString=__new0  BranchType=RL  Resistance=1e-5  Inductance=3.0E-6  SetiL0=off  InitialCurrent=0  Capacitance=1e-6  Setx0=off  InitialVoltage=0  Measurements=None
  Series RLC Branch10 : spsSeriesRLCBranchLib/Series RLC Branch  LConnTagsString=__new0  RConnTagsString=__new0  BranchType=L  Resistance=1  Inductance=0.4e-6  SetiL0=off  InitialCurrent=0  Capacitance=1e-6  Setx0=off  InitialVoltage=0  Measurements=None
  Series RLC Branch12 : spsSeriesRLCBranchLib/Series RLC Branch  LConnTagsString=__new0  RConnTagsString=__new0  BranchType=RL  Resistance=1e-5  Inductance=1E-9  SetiL0=off  InitialCurrent=0  Capacitance=1e-6  Setx0=off  InitialVoltage=0  Measurements=None
  Series RLC Branch14 : spsSeriesRLCBranchLib/Series RLC Branch  LConnTagsString=__new0  RConnTagsString=__new0  BranchType=L  Resistance=1  Inductance=1E-7  SetiL0=off  InitialCurrent=0  Capacitance=1e-6  Setx0=off  InitialVoltage=0  Measurements=None
  Series RLC Branch2 : spsSeriesRLCBranchLib/Series RLC Branch  LConnTagsString=__new0  RConnTagsString=__new0  BranchType=RC  Resistance=1e-5  Inductance=20e-6  SetiL0=off  InitialCurrent=0  Capacitance=17e-6  Setx0=off  InitialVoltage=0  Measurements=None
  Series RLC Branch3 : spsSeriesRLCBranchLib/Series RLC Branch  LConnTagsString=__new0  RConnTagsString=__new0  BranchType=RL  Resistance=1e-5  Inductance=1E-9  SetiL0=off  InitialCurrent=0  Capacitance=1e-6  Setx0=off  InitialVoltage=0  Measurements=None
  Series RLC Branch5 : spsSeriesRLCBranchLib/Series RLC Branch  LConnTagsString=__new0  RConnTagsString=__new0  BranchType=L  Resistance=1  Inductance=1E-7  SetiL0=off  InitialCurrent=0  Capacitance=1e-6  Setx0=off  InitialVoltage=0  Measurements=None
  Series RLC Branch7 : spsSeriesRLCBranchLib/Series RLC Branch  LConnTagsString=__new0  RConnTagsString=__new0  BranchType=RL  Resistance=0.6  Inductance=1e-6  SetiL0=off  InitialCurrent=0  Capacitance=1e-6  Setx0=off  InitialVoltage=0  Measurements=None
  Series RLC Branch9 : spsSeriesRLCBranchLib/Series RLC Branch  LConnTagsString=__new0  RConnTagsString=__new0  BranchType=L  Resistance=1  Inductance=0.4e-6  SetiL0=off  InitialCurrent=0  Capacitance=1e-6  Setx0=off  InitialVoltage=0  Measurements=None
  Terminator{,1..9} (10 alike) : Terminator
  Udc+ : PMIOPort  Side=Left
  udc- : PMIOPort  Port=2  Side=Left
  p1 : PMIOPort  Port=3  Side=Right
  p2 : PMIOPort  Port=4  Side=Right
  wires:
  Diode6/1 -> Terminator1/1
  Diode1/1 -> Terminator6/1
  Diode8/1 -> Terminator7/1
  PWM/1 -> Demux/1
  [p2] -> IGBT/1
  Diode2/1 -> Terminator8/1
  Current Measurement1/1 -> Terminator/1
  [p1] -> IGBT2/1
  [n2] -> IGBT1/1
  IGBT/1 -> Terminator2/1
  IGBT2/1 -> Terminator3/1
  Demux/4 -> [n1]
  Demux/3 -> [n2]
  Demux/2 -> [p1]
  IGBT1/1 -> Terminator4/1
  [n1] -> IGBT3/1
  IGBT3/1 -> Terminator5/1
  Diode3/1 -> Terminator9/1
  Demux/1 -> [p2]
  connections:
  IGBT/RConn1 -- Diode8/LConn1 -- p2/RConn1 -- Diode1/RConn1 -- IGBT1/LConn1
  Series RLC Branch7/LConn1 -- Series RLC Branch1/LConn1 -- Series RLC Branch9/RConn1
  Series RLC Branch14/LConn1 -- Series RLC Branch2/RConn1 -- Series RLC Branch10/RConn1 -- Series RLC Branch5/LConn1
  Diode2/LConn1 -- IGBT2/RConn1 -- IGBT3/LConn1 -- Diode3/RConn1 -- p1/RConn1
  Series RLC Branch12/RConn1 -- IGBT2/LConn1 -- Diode2/RConn1
  Current Measurement1/RConn1 -- Diode6/LConn1
  Series RLC Branch5/RConn1 -- Diode1/LConn1 -- IGBT1/RConn1
  IGBT/LConn1 -- Diode8/RConn1 -- Series RLC Branch3/RConn1
  IGBT3/RConn1 -- Diode3/LConn1 -- Series RLC Branch14/RConn1
  Series RLC Branch1/RConn1 -- Current Measurement1/LConn1 -- Series RLC Branch12/LConn1 -- Series RLC Branch3/LConn1
  Series RLC Branch7/RConn1 -- Diode6/RConn1 -- Series RLC Branch2/LConn1
  Series RLC Branch9/LConn1 -- Udc+/RConn1
  Series RLC Branch10/LConn1 -- udc-/RConn1

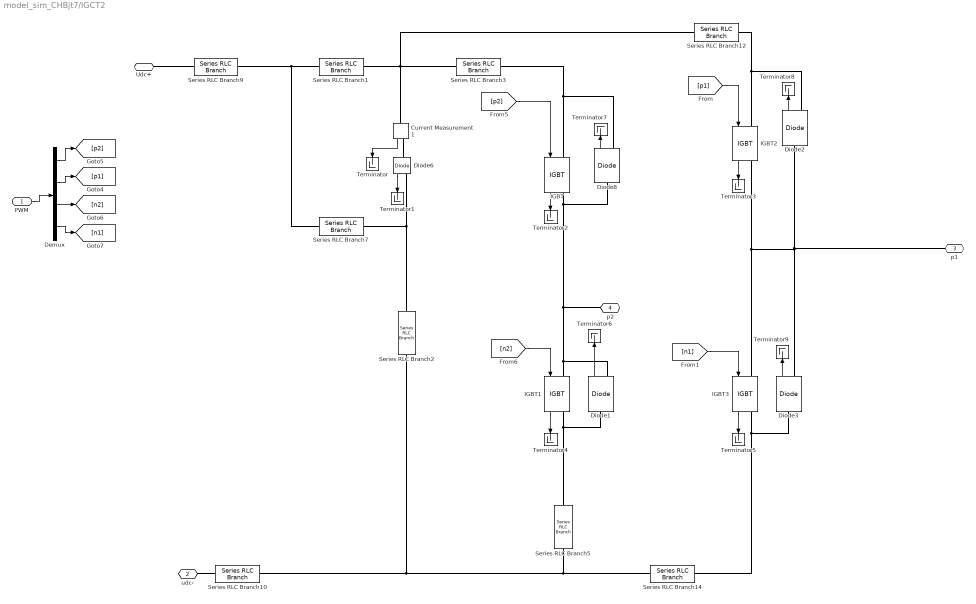
== system model_sim_CHBjt7/IGCT2 ==
  PWM : Inport
  Current Measurement1 : spsCurrentMeasurementLib/Current Measurement  PhasorSimulation=off  OutputType=Complex  PSBequivalent=0
  Demux : Demux
  Diode{1..3,6,8} (5 alike) : spsDiodeLib/Diode  Ron=rto  Lon=0  Vf=vto  IC=0  UseSnubber=off  Rs=500  Cs=250e-9  Measurements=on
  IGBT{,1..3} (4 alike) : spsIGBTLib/IGBT  Ron=rt  Lon=0  Vf=vt  Tf=1e-6  Tt=2e-6  IC=0  Rs=1e5  Cs=inf  Measurements=on
  Series RLC Branch1 : spsSeriesRLCBranchLib/Series RLC Branch  LConnTagsString=__new0  RConnTagsString=__new0  BranchType=RL  Resistance=1e-5  Inductance=3.0E-6  SetiL0=off  InitialCurrent=0  Capacitance=1e-6  Setx0=off  InitialVoltage=0  Measurements=None
  Series RLC Branch10 : spsSeriesRLCBranchLib/Series RLC Branch  LConnTagsString=__new0  RConnTagsString=__new0  BranchType=L  Resistance=1  Inductance=0.4e-6  SetiL0=off  InitialCurrent=0  Capacitance=1e-6  Setx0=off  InitialVoltage=0  Measurements=None
  Series RLC Branch12 : spsSeriesRLCBranchLib/Series RLC Branch  LConnTagsString=__new0  RConnTagsString=__new0  BranchType=RL  Resistance=1e-5  Inductance=1E-9  SetiL0=off  InitialCurrent=0  Capacitance=1e-6  Setx0=off  InitialVoltage=0  Measurements=None
  Series RLC Branch14 : spsSeriesRLCBranchLib/Series RLC Branch  LConnTagsString=__new0  RConnTagsString=__new0  BranchType=L  Resistance=1  Inductance=1E-7  SetiL0=off  InitialCurrent=0  Capacitance=1e-6  Setx0=off  InitialVoltage=0  Measurements=None
  Series RLC Branch2 : spsSeriesRLCBranchLib/Series RLC Branch  LConnTagsString=__new0  RConnTagsString=__new0  BranchType=RC  Resistance=1e-5  Inductance=20e-6  SetiL0=off  InitialCurrent=0  Capacitance=17e-6  Setx0=off  InitialVoltage=0  Measurements=None
  Series RLC Branch3 : spsSeriesRLCBranchLib/Series RLC Branch  LConnTagsString=__new0  RConnTagsString=__new0  BranchType=RL  Resistance=1e-5  Inductance=1E-9  SetiL0=off  InitialCurrent=0  Capacitance=1e-6  Setx0=off  InitialVoltage=0  Measurements=None
  Series RLC Branch5 : spsSeriesRLCBranchLib/Series RLC Branch  LConnTagsString=__new0  RConnTagsString=__new0  BranchType=L  Resistance=1  Inductance=1E-7  SetiL0=off  InitialCurrent=0  Capacitance=1e-6  Setx0=off  InitialVoltage=0  Measurements=None
  Series RLC Branch7 : spsSeriesRLCBranchLib/Series RLC Branch  LConnTagsString=__new0  RConnTagsString=__new0  BranchType=RL  Resistance=0.6  Inductance=1e-6  SetiL0=off  InitialCurrent=0  Capacitance=1e-6  Setx0=off  InitialVoltage=0  Measurements=None
  Series RLC Branch9 : spsSeriesRLCBranchLib/Series RLC Branch  LConnTagsString=__new0  RConnTagsString=__new0  BranchType=L  Resistance=1  Inductance=0.4e-6  SetiL0=off  InitialCurrent=0  Capacitance=1e-6  Setx0=off  InitialVoltage=0  Measurements=None
  Terminator{,1..9} (10 alike) : Terminator
  Udc+ : PMIOPort  Side=Left
  udc- : PMIOPort  Port=2  Side=Left
  p1 : PMIOPort  Port=3  Side=Right
  p2 : PMIOPort  Port=4  Side=Right
  wires:
  Diode3/1 -> Terminator9/1
  IGBT3/1 -> Terminator5/1
  [n1] -> IGBT3/1
  IGBT1/1 -> Terminator4/1
  IGBT2/1 -> Terminator3/1
  IGBT/1 -> Terminator2/1
  [n2] -> IGBT1/1
  [p1] -> IGBT2/1
  Current Measurement1/1 -> Terminator/1
  Diode2/1 -> Terminator8/1
  [p2] -> IGBT/1
  Diode8/1 -> Terminator7/1
  Diode1/1 -> Terminator6/1
  Diode6/1 -> Terminator1/1
  Demux/3 -> [n2]
  PWM/1 -> Demux/1
  Demux/1 -> [p2]
  Demux/2 -> [p1]
  Demux/4 -> [n1]
  connections:
  Series RLC Branch10/LConn1 -- udc-/RConn1
  Series RLC Branch9/LConn1 -- Udc+/RConn1
  Diode6/RConn1 -- Series RLC Branch7/RConn1 -- Series RLC Branch2/LConn1
  Current Measurement1/LConn1 -- Series RLC Branch1/RConn1 -- Series RLC Branch3/LConn1 -- Series RLC Branch12/LConn1
  Diode3/LConn1 -- IGBT3/RConn1 -- Series RLC Branch14/RConn1
  Series RLC Branch3/RConn1 -- IGBT/LConn1 -- Diode8/RConn1
  Diode1/LConn1 -- Series RLC Branch5/RConn1 -- IGBT1/RConn1
  Current Measurement1/RConn1 -- Diode6/LConn1
  Diode2/RConn1 -- Series RLC Branch12/RConn1 -- IGBT2/LConn1
  p1/RConn1 -- Diode2/LConn1 -- Diode3/RConn1 -- IGBT3/LConn1 -- IGBT2/RConn1
  Series RLC Branch5/LConn1 -- Series RLC Branch14/LConn1 -- Series RLC Branch10/RConn1 -- Series RLC Branch2/RConn1
  Series RLC Branch1/LConn1 -- Series RLC Branch7/LConn1 -- Series RLC Branch9/RConn1
  p2/RConn1 -- IGBT1/LConn1 -- Diode1/RConn1 -- Diode8/LConn1 -- IGBT/RConn1

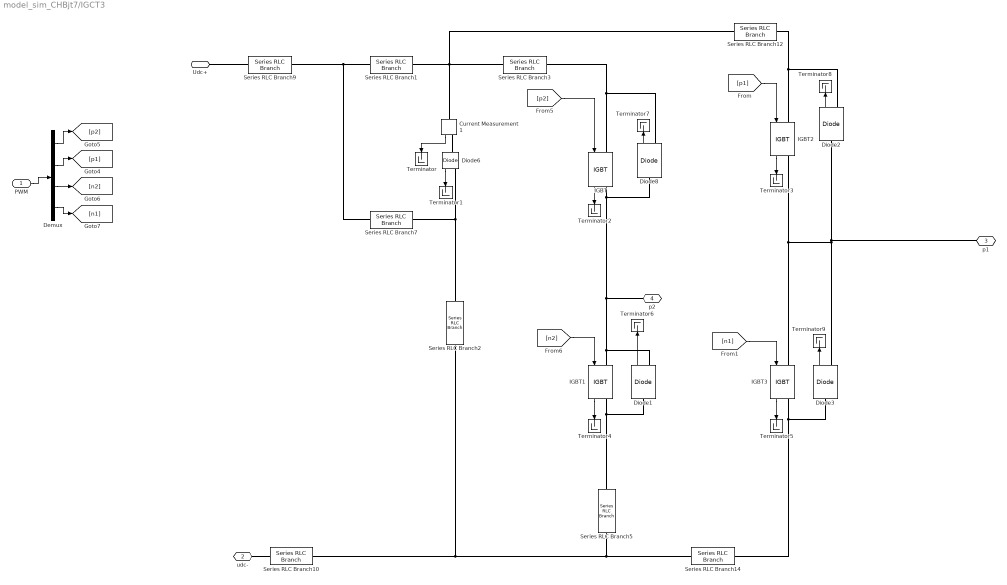
== system model_sim_CHBjt7/IGCT3 ==
  PWM : Inport
  Current Measurement1 : spsCurrentMeasurementLib/Current Measurement  PhasorSimulation=off  OutputType=Complex  PSBequivalent=0
  Demux : Demux
  Diode{1..3,6,8} (5 alike) : spsDiodeLib/Diode  Ron=rto  Lon=0  Vf=vto  IC=0  UseSnubber=off  Rs=500  Cs=250e-9  Measurements=on
  IGBT{,1..3} (4 alike) : spsIGBTLib/IGBT  Ron=rt  Lon=0  Vf=vt  Tf=1e-6  Tt=2e-6  IC=0  Rs=1e5  Cs=inf  Measurements=on
  Series RLC Branch1 : spsSeriesRLCBranchLib/Series RLC Branch  LConnTagsString=__new0  RConnTagsString=__new0  BranchType=RL  Resistance=1e-5  Inductance=3.0E-6  SetiL0=off  InitialCurrent=0  Capacitance=1e-6  Setx0=off  InitialVoltage=0  Measurements=None
  Series RLC Branch10 : spsSeriesRLCBranchLib/Series RLC Branch  LConnTagsString=__new0  RConnTagsString=__new0  BranchType=L  Resistance=1  Inductance=0.4e-6  SetiL0=off  InitialCurrent=0  Capacitance=1e-6  Setx0=off  InitialVoltage=0  Measurements=None
  Series RLC Branch12 : spsSeriesRLCBranchLib/Series RLC Branch  LConnTagsString=__new0  RConnTagsString=__new0  BranchType=RL  Resistance=1e-5  Inductance=1E-9  SetiL0=off  InitialCurrent=0  Capacitance=1e-6  Setx0=off  InitialVoltage=0  Measurements=None
  Series RLC Branch14 : spsSeriesRLCBranchLib/Series RLC Branch  LConnTagsString=__new0  RConnTagsString=__new0  BranchType=L  Resistance=1  Inductance=1E-7  SetiL0=off  InitialCurrent=0  Capacitance=1e-6  Setx0=off  InitialVoltage=0  Measurements=None
  Series RLC Branch2 : spsSeriesRLCBranchLib/Series RLC Branch  LConnTagsString=__new0  RConnTagsString=__new0  BranchType=RC  Resistance=1e-5  Inductance=20e-6  SetiL0=off  InitialCurrent=0  Capacitance=17e-6  Setx0=off  InitialVoltage=0  Measurements=None
  Series RLC Branch3 : spsSeriesRLCBranchLib/Series RLC Branch  LConnTagsString=__new0  RConnTagsString=__new0  BranchType=RL  Resistance=1e-5  Inductance=1E-9  SetiL0=off  InitialCurrent=0  Capacitance=1e-6  Setx0=off  InitialVoltage=0  Measurements=None
  Series RLC Branch5 : spsSeriesRLCBranchLib/Series RLC Branch  LConnTagsString=__new0  RConnTagsString=__new0  BranchType=L  Resistance=1  Inductance=1E-7  SetiL0=off  InitialCurrent=0  Capacitance=1e-6  Setx0=off  InitialVoltage=0  Measurements=None
  Series RLC Branch7 : spsSeriesRLCBranchLib/Series RLC Branch  LConnTagsString=__new0  RConnTagsString=__new0  BranchType=RL  Resistance=0.6  Inductance=1e-6  SetiL0=off  InitialCurrent=0  Capacitance=1e-6  Setx0=off  InitialVoltage=0  Measurements=None
  Series RLC Branch9 : spsSeriesRLCBranchLib/Series RLC Branch  LConnTagsString=__new0  RConnTagsString=__new0  BranchType=L  Resistance=1  Inductance=0.4e-6  SetiL0=off  InitialCurrent=0  Capacitance=1e-6  Setx0=off  InitialVoltage=0  Measurements=None
  Terminator{,1..9} (10 alike) : Terminator
  Udc+ : PMIOPort  Side=Left
  udc- : PMIOPort  Port=2  Side=Left
  p1 : PMIOPort  Port=3  Side=Right
  p2 : PMIOPort  Port=4  Side=Right
  wires:
  Diode3/1 -> Terminator9/1
  IGBT3/1 -> Terminator5/1
  [n1] -> IGBT3/1
  IGBT1/1 -> Terminator4/1
  IGBT2/1 -> Terminator3/1
  IGBT/1 -> Terminator2/1
  [n2] -> IGBT1/1
  [p1] -> IGBT2/1
  Current Measurement1/1 -> Terminator/1
  Diode2/1 -> Terminator8/1
  [p2] -> IGBT/1
  Diode8/1 -> Terminator7/1
  Diode1/1 -> Terminator6/1
  Diode6/1 -> Terminator1/1
  Demux/3 -> [n2]
  PWM/1 -> Demux/1
  Demux/1 -> [p2]
  Demux/2 -> [p1]
  Demux/4 -> [n1]
  connections:
  Series RLC Branch10/LConn1 -- udc-/RConn1
  Series RLC Branch9/LConn1 -- Udc+/RConn1
  Diode6/RConn1 -- Series RLC Branch7/RConn1 -- Series RLC Branch2/LConn1
  Current Measurement1/LConn1 -- Series RLC Branch1/RConn1 -- Series RLC Branch3/LConn1 -- Series RLC Branch12/LConn1
  Diode3/LConn1 -- IGBT3/RConn1 -- Series RLC Branch14/RConn1
  Series RLC Branch3/RConn1 -- IGBT/LConn1 -- Diode8/RConn1
  Diode1/LConn1 -- Series RLC Branch5/RConn1 -- IGBT1/RConn1
  Current Measurement1/RConn1 -- Diode6/LConn1
  Diode2/RConn1 -- Series RLC Branch12/RConn1 -- IGBT2/LConn1
  p1/RConn1 -- Diode2/LConn1 -- Diode3/RConn1 -- IGBT3/LConn1 -- IGBT2/RConn1
  Series RLC Branch5/LConn1 -- Series RLC Branch14/LConn1 -- Series RLC Branch10/RConn1 -- Series RLC Branch2/RConn1
  Series RLC Branch1/LConn1 -- Series RLC Branch7/LConn1 -- Series RLC Branch9/RConn1
  p2/RConn1 -- IGBT1/LConn1 -- Diode1/RConn1 -- Diode8/LConn1 -- IGBT/RConn1

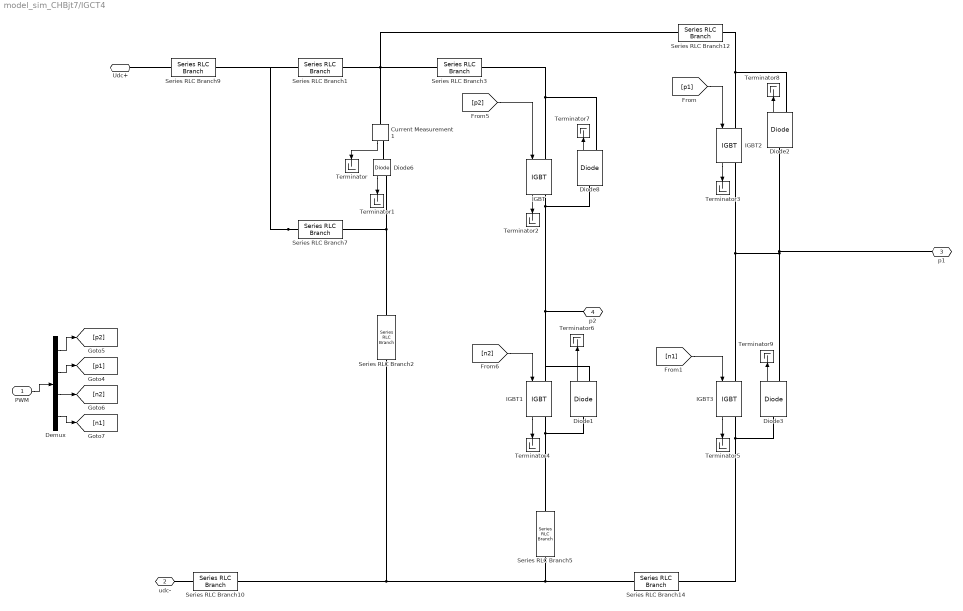
== system model_sim_CHBjt7/IGCT4 ==
  PWM : Inport
  Current Measurement1 : spsCurrentMeasurementLib/Current Measurement  PhasorSimulation=off  OutputType=Complex  PSBequivalent=0
  Demux : Demux
  Diode{1..3,6,8} (5 alike) : spsDiodeLib/Diode  Ron=rto  Lon=0  Vf=vto  IC=0  UseSnubber=off  Rs=500  Cs=250e-9  Measurements=on
  IGBT{,1..3} (4 alike) : spsIGBTLib/IGBT  Ron=rt  Lon=0  Vf=vt  Tf=1e-6  Tt=2e-6  IC=0  Rs=1e5  Cs=inf  Measurements=on
  Series RLC Branch1 : spsSeriesRLCBranchLib/Series RLC Branch  LConnTagsString=__new0  RConnTagsString=__new0  BranchType=RL  Resistance=1e-5  Inductance=3.0E-6  SetiL0=off  InitialCurrent=0  Capacitance=1e-6  Setx0=off  InitialVoltage=0  Measurements=None
  Series RLC Branch10 : spsSeriesRLCBranchLib/Series RLC Branch  LConnTagsString=__new0  RConnTagsString=__new0  BranchType=L  Resistance=1  Inductance=0.4e-6  SetiL0=off  InitialCurrent=0  Capacitance=1e-6  Setx0=off  InitialVoltage=0  Measurements=None
  Series RLC Branch12 : spsSeriesRLCBranchLib/Series RLC Branch  LConnTagsString=__new0  RConnTagsString=__new0  BranchType=RL  Resistance=1e-5  Inductance=1E-9  SetiL0=off  InitialCurrent=0  Capacitance=1e-6  Setx0=off  InitialVoltage=0  Measurements=None
  Series RLC Branch14 : spsSeriesRLCBranchLib/Series RLC Branch  LConnTagsString=__new0  RConnTagsString=__new0  BranchType=L  Resistance=1  Inductance=1E-7  SetiL0=off  InitialCurrent=0  Capacitance=1e-6  Setx0=off  InitialVoltage=0  Measurements=None
  Series RLC Branch2 : spsSeriesRLCBranchLib/Series RLC Branch  LConnTagsString=__new0  RConnTagsString=__new0  BranchType=RC  Resistance=1e-5  Inductance=20e-6  SetiL0=off  InitialCurrent=0  Capacitance=17e-6  Setx0=off  InitialVoltage=0  Measurements=None
  Series RLC Branch3 : spsSeriesRLCBranchLib/Series RLC Branch  LConnTagsString=__new0  RConnTagsString=__new0  BranchType=RL  Resistance=1e-5  Inductance=1E-9  SetiL0=off  InitialCurrent=0  Capacitance=1e-6  Setx0=off  InitialVoltage=0  Measurements=None
  Series RLC Branch5 : spsSeriesRLCBranchLib/Series RLC Branch  LConnTagsString=__new0  RConnTagsString=__new0  BranchType=L  Resistance=1  Inductance=1E-7  SetiL0=off  InitialCurrent=0  Capacitance=1e-6  Setx0=off  InitialVoltage=0  Measurements=None
  Series RLC Branch7 : spsSeriesRLCBranchLib/Series RLC Branch  LConnTagsString=__new0  RConnTagsString=__new0  BranchType=RL  Resistance=0.6  Inductance=1e-6  SetiL0=off  InitialCurrent=0  Capacitance=1e-6  Setx0=off  InitialVoltage=0  Measurements=None
  Series RLC Branch9 : spsSeriesRLCBranchLib/Series RLC Branch  LConnTagsString=__new0  RConnTagsString=__new0  BranchType=L  Resistance=1  Inductance=0.4e-6  SetiL0=off  InitialCurrent=0  Capacitance=1e-6  Setx0=off  InitialVoltage=0  Measurements=None
  Terminator{,1..9} (10 alike) : Terminator
  Udc+ : PMIOPort  Side=Left
  udc- : PMIOPort  Port=2  Side=Left
  p1 : PMIOPort  Port=3  Side=Right
  p2 : PMIOPort  Port=4  Side=Right
  wires:
  Diode6/1 -> Terminator1/1
  Diode1/1 -> Terminator6/1
  Diode8/1 -> Terminator7/1
  PWM/1 -> Demux/1
  [p2] -> IGBT/1
  Diode2/1 -> Terminator8/1
  Current Measurement1/1 -> Terminator/1
  [p1] -> IGBT2/1
  [n2] -> IGBT1/1
  IGBT/1 -> Terminator2/1
  IGBT2/1 -> Terminator3/1
  Demux/4 -> [n1]
  Demux/3 -> [n2]
  Demux/2 -> [p1]
  IGBT1/1 -> Terminator4/1
  [n1] -> IGBT3/1
  IGBT3/1 -> Terminator5/1
  Diode3/1 -> Terminator9/1
  Demux/1 -> [p2]
  connections:
  IGBT/RConn1 -- Diode8/LConn1 -- p2/RConn1 -- Diode1/RConn1 -- IGBT1/LConn1
  Series RLC Branch7/LConn1 -- Series RLC Branch1/LConn1 -- Series RLC Branch9/RConn1
  Series RLC Branch14/LConn1 -- Series RLC Branch2/RConn1 -- Series RLC Branch10/RConn1 -- Series RLC Branch5/LConn1
  Diode2/LConn1 -- IGBT2/RConn1 -- IGBT3/LConn1 -- Diode3/RConn1 -- p1/RConn1
  Series RLC Branch12/RConn1 -- IGBT2/LConn1 -- Diode2/RConn1
  Current Measurement1/RConn1 -- Diode6/LConn1
  Series RLC Branch5/RConn1 -- Diode1/LConn1 -- IGBT1/RConn1
  IGBT/LConn1 -- Diode8/RConn1 -- Series RLC Branch3/RConn1
  IGBT3/RConn1 -- Diode3/LConn1 -- Series RLC Branch14/RConn1
  Series RLC Branch1/RConn1 -- Current Measurement1/LConn1 -- Series RLC Branch12/LConn1 -- Series RLC Branch3/LConn1
  Series RLC Branch7/RConn1 -- Diode6/RConn1 -- Series RLC Branch2/LConn1
  Series RLC Branch9/LConn1 -- Udc+/RConn1
  Series RLC Branch10/LConn1 -- udc-/RConn1
